simulink model "TesteControle"  (R2024a)
settings: Solver=ode4  StartTime=0.0  StopTime=10.0  FixedStep=1/100  RelTol=1e-3
settings Model: Creator=igmso  LastModifiedBy=igmso
settings SFSimCC: SimCustomHeaderCode="#include \"gnc.h\""  SimTargetLang=C++
settings SFSimCC: SimUserSources=|
  | math_utils.c
  | pid.c
  | atp.c
  | gnc.c
settings SFSimCC: SimUserIncludeDirs=|
  | C:\Users\igmso\Desktop\Tilt\C\lib
  | C:\Users\igmso\Desktop\Tilt\C\src

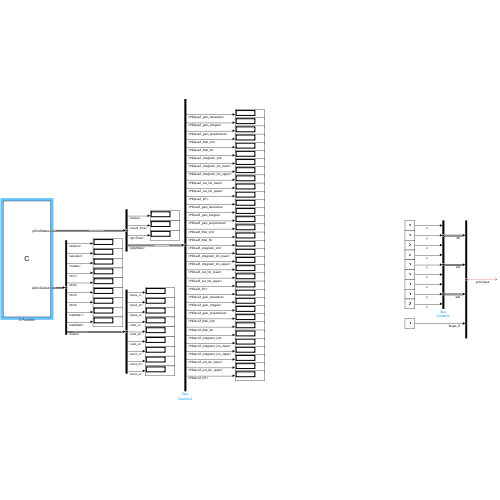
[thumbnail: Simulink's stored preview of the top-level diagram]
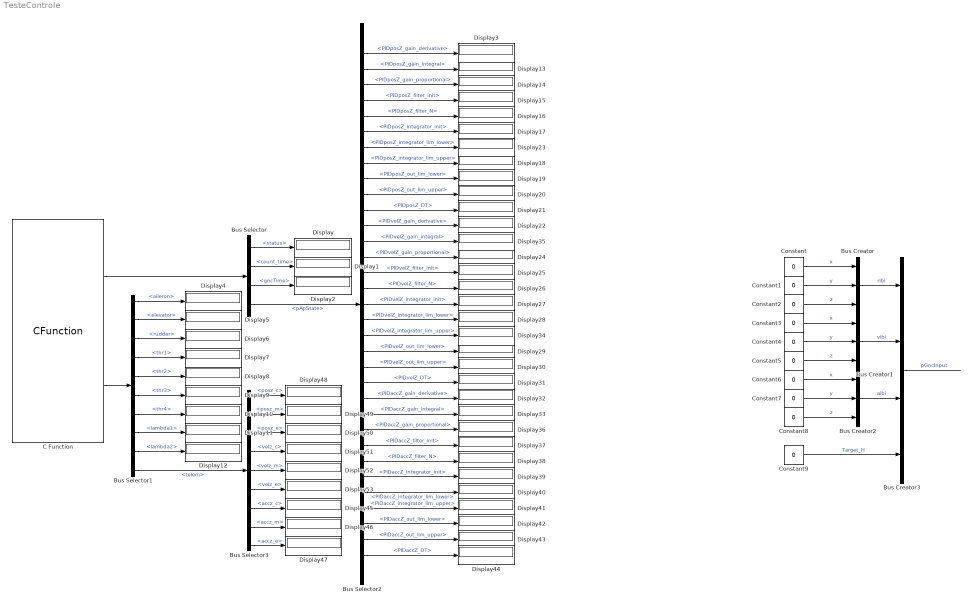
== system TesteControle ==
  Bus Creator : BusCreator  Inputs=3
  Bus Creator1 : BusCreator  Inputs=3
  Bus Creator2 : BusCreator  Inputs=3
  Bus Creator3 : BusCreator  Inputs=4
  Bus Selector : BusSelector  OutputSignals=status,count_time,gncTime,pApState
  Bus Selector1 : BusSelector  OutputSignals=aileron,elevator,rudder,thr1,thr2,thr3,thr4,lambda1,lambda2,telem
  Bus Selector2 : BusSelector  OutputSignals=PIDposZ_gain_derivative,PIDposZ_gain_integral,PIDposZ_gain_proportional,PIDposZ_filter_init,PIDposZ_filter_N,PIDposZ_integrator_init,PIDposZ_integrator_lim_lower,PIDposZ_integrator_lim_upper,PIDposZ_out_lim_lower,PIDposZ_out_lim_upper,PIDposZ_DT,PIDvelZ_gain_derivative,PIDvelZ_gain_integral,PIDvelZ_gain_proportional,PIDvelZ_filter_init,PIDvelZ_filter_N,PIDvelZ_integrator_init,PIDvelZ_integrator_lim_lower,PIDvelZ_integrator_lim_upper,PIDvelZ_out_lim_lower,PIDvelZ_out_lim_upper,PIDvelZ_DT,PIDaccZ_gain_derivative,PIDaccZ_gain_integral,PIDaccZ_gain_proportional,PIDaccZ_filter_init,PIDaccZ_filter_N,PIDaccZ_integrator_init,PIDaccZ_integrator_lim_lower,PIDaccZ_integrator_lim_upper,PIDaccZ_out_lim_lower,PIDaccZ_out_lim_upper,PIDaccZ_DT
  Bus Selector3 : BusSelector  OutputSignals=posz_c,posz_m,posz_e,velz_c,velz_m,velz_e,accz_c,accz_m,accz_e
  C Function : CFunction  OutputCode=|  CodegenOutputCode=|
      OutputCode=|
      | /* Initialization
      | void GNC_Init(GNC_State_t *pGncStates, GNC_Output_t *pGncOutput)
      | */
      | GNC_Init(&pGncStates,&pGncOutput);
      CodegenOutputCode=|
      | /* Initialization
      | void GNC_Init(GNC_State_t *pGncStates, GNC_Output_t *pGncOutput)
      | */
      | GNC_Init(&pGncStates,&pGncOutput);
  Constant{,1..9} (10 alike) : Constant  Value=0  SampleTime=-1
  Display{,1..53} (54 alike) : Display
  wires:
  Constant/1 -> Bus Creator/1  "x"
  Constant1/1 -> Bus Creator/2  "y"
  Constant2/1 -> Bus Creator/3  "z"
  Bus Creator/1 -> Bus Creator3/1  "ribi"
  Bus Creator1/1 -> Bus Creator3/2  "vibi"
  Constant5/1 -> Bus Creator1/3  "z"
  Constant4/1 -> Bus Creator1/2  "y"
  Constant3/1 -> Bus Creator1/1  "x"
  Constant6/1 -> Bus Creator2/1  "x"
  Constant7/1 -> Bus Creator2/2  "y"
  Constant8/1 -> Bus Creator2/3  "z"
  Bus Creator2/1 -> Bus Creator3/3  "aibi"
  Constant9/1 -> Bus Creator3/4  "Target_H"
  Bus Creator3/1 -> ?  "pGncInput"
  C Function/1 -> Bus Selector/1
  Bus Selector/4 -> Bus Selector2/1  "<pApState>"
  Bus Selector/3 -> Display2/1  "<gncTime>"
  Bus Selector/2 -> Display1/1  "<count_time>"
  Bus Selector/1 -> Display/1  "<status>"
  C Function/2 -> Bus Selector1/1
  Bus Selector1/1 -> Display4/1  "<aileron>"
  Bus Selector1/2 -> Display5/1  "<elevator>"
  Bus Selector1/3 -> Display6/1  "<rudder>"
  Bus Selector1/4 -> Display7/1  "<thr1>"
  Bus Selector1/7 -> Display10/1  "<thr4>"
  Bus Selector1/6 -> Display9/1  "<thr3>"
  Bus Selector1/5 -> Display8/1  "<thr2>"
  Bus Selector1/8 -> Display11/1  "<lambda1>"
  Bus Selector1/9 -> Display12/1  "<lambda2>"
  Bus Selector1/10 -> Bus Selector3/1  "<telem>"
  Bus Selector2/1 -> Display3/1  "<PIDposZ_gain_derivative>"
  Bus Selector2/2 -> Display13/1  "<PIDposZ_gain_integral>"
  Bus Selector2/3 -> Display14/1  "<PIDposZ_gain_proportional>"
  Bus Selector2/4 -> Display15/1  "<PIDposZ_filter_init>"
  Bus Selector2/5 -> Display16/1  "<PIDposZ_filter_N>"
  Bus Selector2/6 -> Display17/1  "<PIDposZ_integrator_init>"
  Bus Selector2/7 -> Display23/1  "<PIDposZ_integrator_lim_lower>"
  Bus Selector2/8 -> Display18/1  "<PIDposZ_integrator_lim_upper>"
  Bus Selector2/9 -> Display19/1  "<PIDposZ_out_lim_lower>"
  Bus Selector2/10 -> Display20/1  "<PIDposZ_out_lim_upper>"
  Bus Selector2/11 -> Display21/1  "<PIDposZ_DT>"
  Bus Selector2/12 -> Display22/1  "<PIDvelZ_gain_derivative>"
  Bus Selector2/13 -> Display35/1  "<PIDvelZ_gain_integral>"
  Bus Selector2/14 -> Display24/1  "<PIDvelZ_gain_proportional>"
  Bus Selector2/15 -> Display25/1  "<PIDvelZ_filter_init>"
  Bus Selector2/16 -> Display26/1  "<PIDvelZ_filter_N>"
  Bus Selector2/17 -> Display27/1  "<PIDvelZ_integrator_init>"
  Bus Selector2/18 -> Display28/1  "<PIDvelZ_integrator_lim_lower>"
  Bus Selector2/19 -> Display34/1  "<PIDvelZ_integrator_lim_upper>"
  Bus Selector2/20 -> Display29/1  "<PIDvelZ_out_lim_lower>"
  Bus Selector2/21 -> Display30/1  "<PIDvelZ_out_lim_upper>"
  Bus Selector2/22 -> Display31/1  "<PIDvelZ_DT>"
  Bus Selector2/23 -> Display32/1  "<PIDaccZ_gain_derivative>"
  Bus Selector2/24 -> Display33/1  "<PIDaccZ_gain_integral>"
  Bus Selector2/25 -> Display36/1  "<PIDaccZ_gain_proportional>"
  Bus Selector2/26 -> Display37/1  "<PIDaccZ_filter_init>"
  Bus Selector2/27 -> Display38/1  "<PIDaccZ_filter_N>"
  Bus Selector2/28 -> Display39/1  "<PIDaccZ_integrator_init>"
  Bus Selector2/29 -> Display40/1  "<PIDaccZ_integrator_lim_lower>"
  Bus Selector2/30 -> Display41/1  "<PIDaccZ_integrator_lim_upper>"
  Bus Selector2/31 -> Display42/1  "<PIDaccZ_out_lim_lower>"
  Bus Selector2/32 -> Display43/1  "<PIDaccZ_out_lim_upper>"
  Bus Selector2/33 -> Display44/1  "<PIDaccZ_DT>"
  Bus Selector3/1 -> Display48/1  "<posz_c>"
  Bus Selector3/2 -> Display49/1  "<posz_m>"
  Bus Selector3/3 -> Display50/1  "<posz_e>"
  Bus Selector3/4 -> Display51/1  "<velz_c>"
  Bus Selector3/5 -> Display52/1  "<velz_m>"
  Bus Selector3/6 -> Display53/1  "<velz_e>"
  Bus Selector3/7 -> Display45/1  "<accz_c>"
  Bus Selector3/8 -> Display46/1  "<accz_m>"
  Bus Selector3/9 -> Display47/1  "<accz_e>"
